simulink library "ReceiveFromGES"  (R2016b)
settings: Solver=VariableStepAuto  StartTime=0.0  StopTime=10.0  RelTol=1e-3
libraries: xpcethercatlib x12, ReceiveFromGES x3, simulink_extras x3, VariousLibrary x1
settings Model: Creator=Nathan  LastModifiedBy=march

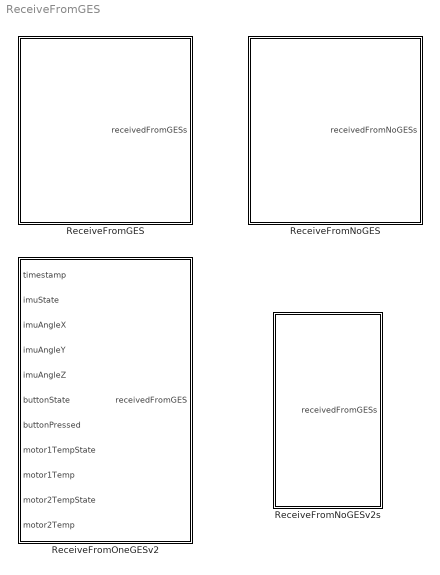
== system ReceiveFromGES ==
  ReceiveFromGES : Subsystem
  ReceiveFromNoGES : Subsystem
  ReceiveFromNoGESv2s : Subsystem
  ReceiveFromOneGESv2 : Subsystem

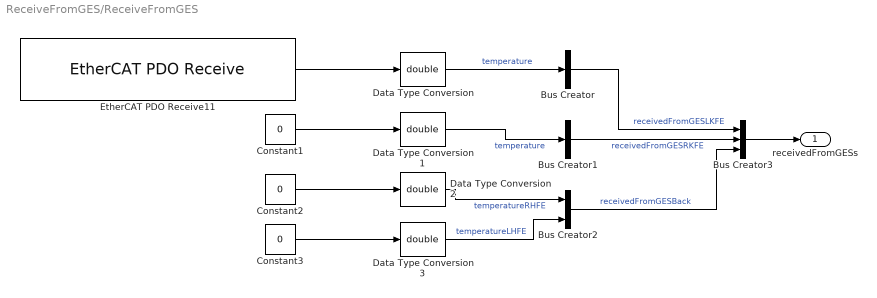
== system ReceiveFromGES/ReceiveFromGES ==
  Bus Creator : BusCreator  Inputs=1  OutDataTypeStr=Bus: EtherCATReceivedFromGESJoint  NonVirtualBus=on
  Bus Creator1 : BusCreator  Inputs=1  OutDataTypeStr=Bus: EtherCATReceivedFromGESJoint  NonVirtualBus=on
  Bus Creator2 : BusCreator  Inputs=2  OutDataTypeStr=Bus: EtherCATReceivedFromGESBack  NonVirtualBus=on
  Bus Creator3 : BusCreator  Inputs=3  OutDataTypeStr=Bus: EtherCATReceivedFromGES  NonVirtualBus=on
  Constant1 : Constant  Value=0
  Constant2 : Constant  Value=0
  Constant3 : Constant  Value=0
  Data Type Conversion{,1..3} (4 alike) : DataTypeConversion  OutDataTypeStr=double
  EtherCAT PDO Receive11 : xpcethercatlib/EtherCAT PDO Receive  Priority=2  sig_name=Box 2 (EasyCAT 32+32 configurable PDO).Inputs.temperature  sig_offset=728  sig_type=single  type_size=32  sig_dim=1  device_id=0  sample_time=0.002000
  receivedFromGESs : Outport  OutDataTypeStr=Bus: EtherCATReceivedFromGES
  wires:
  Data Type Conversion3/1 -> Bus Creator2/2  "temperatureLHFE"
  Bus Creator3/1 -> receivedFromGESs/1
  Bus Creator/1 -> Bus Creator3/1  "receivedFromGESLKFE"
  Bus Creator2/1 -> Bus Creator3/3  "receivedFromGESBack"
  Bus Creator1/1 -> Bus Creator3/2  "receivedFromGESRKFE"
  Data Type Conversion/1 -> Bus Creator/1  "temperature"
  Data Type Conversion2/1 -> Bus Creator2/1  "temperatureRHFE"
  Data Type Conversion1/1 -> Bus Creator1/1  "temperature"
  Constant1/1 -> Data Type Conversion1/1
  Constant2/1 -> Data Type Conversion2/1
  Constant3/1 -> Data Type Conversion3/1
  EtherCAT PDO Receive11/1 -> Data Type Conversion/1

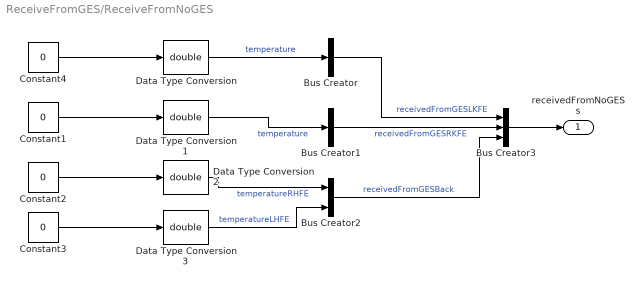
== system ReceiveFromGES/ReceiveFromNoGES ==
  Bus Creator : BusCreator  Inputs=1  OutDataTypeStr=Bus: EtherCATReceivedFromGESJoint  NonVirtualBus=on
  Bus Creator1 : BusCreator  Inputs=1  OutDataTypeStr=Bus: EtherCATReceivedFromGESJoint  NonVirtualBus=on
  Bus Creator2 : BusCreator  Inputs=2  OutDataTypeStr=Bus: EtherCATReceivedFromGESBack  NonVirtualBus=on
  Bus Creator3 : BusCreator  Inputs=3  OutDataTypeStr=Bus: EtherCATReceivedFromGES  NonVirtualBus=on
  Constant{1..4} (4 alike) : Constant  Value=0
  Data Type Conversion{,1..3} (4 alike) : DataTypeConversion  OutDataTypeStr=double
  receivedFromNoGESs : Outport  OutDataTypeStr=Bus: EtherCATReceivedFromGES
  wires:
  Constant4/1 -> Data Type Conversion/1
  Constant3/1 -> Data Type Conversion3/1
  Constant2/1 -> Data Type Conversion2/1
  Constant1/1 -> Data Type Conversion1/1
  Data Type Conversion1/1 -> Bus Creator1/1  "temperature"
  Data Type Conversion2/1 -> Bus Creator2/1  "temperatureRHFE"
  Data Type Conversion/1 -> Bus Creator/1  "temperature"
  Bus Creator1/1 -> Bus Creator3/2  "receivedFromGESRKFE"
  Bus Creator2/1 -> Bus Creator3/3  "receivedFromGESBack"
  Bus Creator/1 -> Bus Creator3/1  "receivedFromGESLKFE"
  Bus Creator3/1 -> receivedFromNoGESs/1
  Data Type Conversion3/1 -> Bus Creator2/2  "temperatureLHFE"

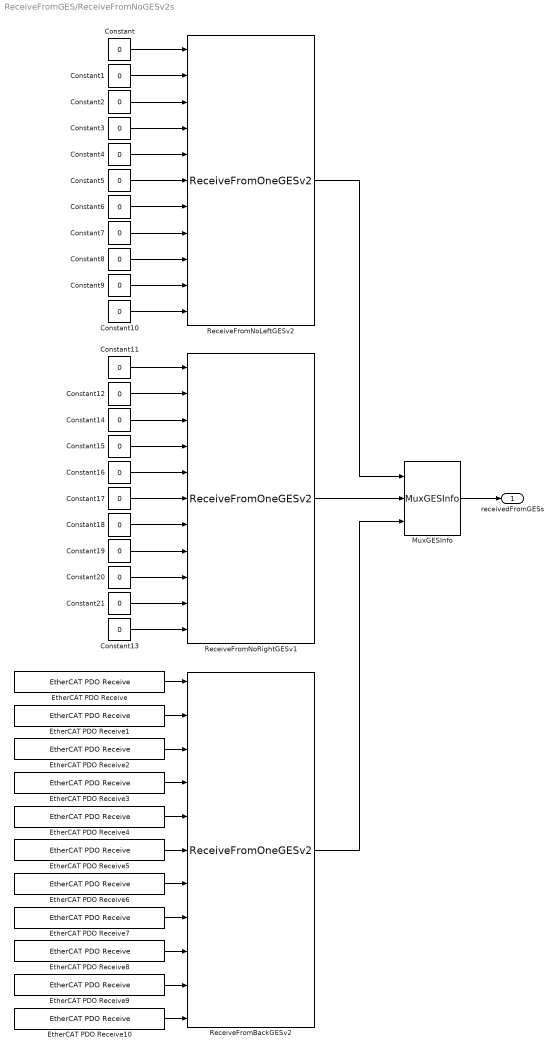
== system ReceiveFromGES/ReceiveFromNoGESv2s ==
  Constant{,1..21} (22 alike) : Constant  Value=0
  EtherCAT PDO Receive : xpcethercatlib/EtherCAT PDO Receive  Priority=2  sig_name=GES Buzzer.Inputs.heartbeat  sig_offset=632  sig_type=uint8  type_size=8  sig_dim=1  device_id=0  sample_time=0.002
  EtherCAT PDO Receive1 : xpcethercatlib/EtherCAT PDO Receive  Priority=2  sig_name=GES Buzzer.Inputs.imuEnabled  sig_offset=640  sig_type=uint8  type_size=8  sig_dim=1  device_id=0  sample_time=0.002
  EtherCAT PDO Receive10 : xpcethercatlib/EtherCAT PDO Receive  Priority=2  sig_name=GES Buzzer.Inputs.motor2Temp  sig_offset=712  sig_type=uint8  type_size=8  sig_dim=1  device_id=0  sample_time=0.002
  EtherCAT PDO Receive2 : xpcethercatlib/EtherCAT PDO Receive  Priority=2  sig_name=GES Buzzer.Inputs.imuAngleX  sig_offset=648  sig_type=uint8  type_size=8  sig_dim=1  device_id=0  sample_time=0.002
  EtherCAT PDO Receive3 : xpcethercatlib/EtherCAT PDO Receive  Priority=2  sig_name=GES Buzzer.Inputs.imuAngleY  sig_offset=656  sig_type=uint8  type_size=8  sig_dim=1  device_id=0  sample_time=0.002
  EtherCAT PDO Receive4 : xpcethercatlib/EtherCAT PDO Receive  Priority=2  sig_name=GES Buzzer.Inputs.imuAngleZ  sig_offset=664  sig_type=uint8  type_size=8  sig_dim=1  device_id=0  sample_time=0.002
  EtherCAT PDO Receive5 : xpcethercatlib/EtherCAT PDO Receive  Priority=2  sig_name=GES Buzzer.Inputs.buttonEnabled  sig_offset=672  sig_type=uint8  type_size=8  sig_dim=1  device_id=0  sample_time=0.002
  EtherCAT PDO Receive6 : xpcethercatlib/EtherCAT PDO Receive  Priority=2  sig_name=GES Buzzer.Inputs.buttonState  sig_offset=680  sig_type=uint8  type_size=8  sig_dim=1  device_id=0  sample_time=0.002
  EtherCAT PDO Receive7 : xpcethercatlib/EtherCAT PDO Receive  Priority=2  sig_name=GES Buzzer.Inputs.motor1TempEnabled  sig_offset=688  sig_type=uint8  type_size=8  sig_dim=1  device_id=0  sample_time=0.002
  EtherCAT PDO Receive8 : xpcethercatlib/EtherCAT PDO Receive  Priority=2  sig_name=GES Buzzer.Inputs.motor1Temp  sig_offset=704  sig_type=uint8  type_size=8  sig_dim=1  device_id=0  sample_time=0.002
  EtherCAT PDO Receive9 : xpcethercatlib/EtherCAT PDO Receive  Priority=2  sig_name=GES Buzzer.Inputs.motor2TempEnabled  sig_offset=696  sig_type=uint8  type_size=8  sig_dim=1  device_id=0  sample_time=0.002
  MuxGESInfo : VariousLibrary/MuxGESInfo
  ReceiveFromBackGESv2 : ReceiveFromGES/ReceiveFromOneGESv2
  ReceiveFromNoLeftGESv2 : ReceiveFromGES/ReceiveFromOneGESv2
  ReceiveFromNoRightGESv1 : ReceiveFromGES/ReceiveFromOneGESv2
  receivedFromGESs : Outport
  wires:
  EtherCAT PDO Receive10/1 -> ReceiveFromBackGESv2/11
  EtherCAT PDO Receive9/1 -> ReceiveFromBackGESv2/10
  EtherCAT PDO Receive8/1 -> ReceiveFromBackGESv2/9
  EtherCAT PDO Receive7/1 -> ReceiveFromBackGESv2/8
  EtherCAT PDO Receive6/1 -> ReceiveFromBackGESv2/7
  EtherCAT PDO Receive5/1 -> ReceiveFromBackGESv2/6
  EtherCAT PDO Receive4/1 -> ReceiveFromBackGESv2/5
  EtherCAT PDO Receive3/1 -> ReceiveFromBackGESv2/4
  EtherCAT PDO Receive2/1 -> ReceiveFromBackGESv2/3
  EtherCAT PDO Receive1/1 -> ReceiveFromBackGESv2/2
  EtherCAT PDO Receive/1 -> ReceiveFromBackGESv2/1
  Constant/1 -> ReceiveFromNoLeftGESv2/1
  Constant1/1 -> ReceiveFromNoLeftGESv2/2
  Constant4/1 -> ReceiveFromNoLeftGESv2/5
  Constant2/1 -> ReceiveFromNoLeftGESv2/3
  Constant5/1 -> ReceiveFromNoLeftGESv2/6
  Constant10/1 -> ReceiveFromNoLeftGESv2/11
  Constant7/1 -> ReceiveFromNoLeftGESv2/8
  Constant3/1 -> ReceiveFromNoLeftGESv2/4
  Constant6/1 -> ReceiveFromNoLeftGESv2/7
  Constant8/1 -> ReceiveFromNoLeftGESv2/9
  Constant9/1 -> ReceiveFromNoLeftGESv2/10
  Constant11/1 -> ReceiveFromNoRightGESv1/1
  Constant12/1 -> ReceiveFromNoRightGESv1/2
  Constant16/1 -> ReceiveFromNoRightGESv1/5
  Constant14/1 -> ReceiveFromNoRightGESv1/3
  Constant17/1 -> ReceiveFromNoRightGESv1/6
  Constant13/1 -> ReceiveFromNoRightGESv1/11
  Constant19/1 -> ReceiveFromNoRightGESv1/8
  Constant15/1 -> ReceiveFromNoRightGESv1/4
  Constant18/1 -> ReceiveFromNoRightGESv1/7
  Constant20/1 -> ReceiveFromNoRightGESv1/9
  Constant21/1 -> ReceiveFromNoRightGESv1/10
  ReceiveFromNoRightGESv1/1 -> MuxGESInfo/2
  ReceiveFromNoLeftGESv2/1 -> MuxGESInfo/1
  ReceiveFromBackGESv2/1 -> MuxGESInfo/3
  MuxGESInfo/1 -> receivedFromGESs/1

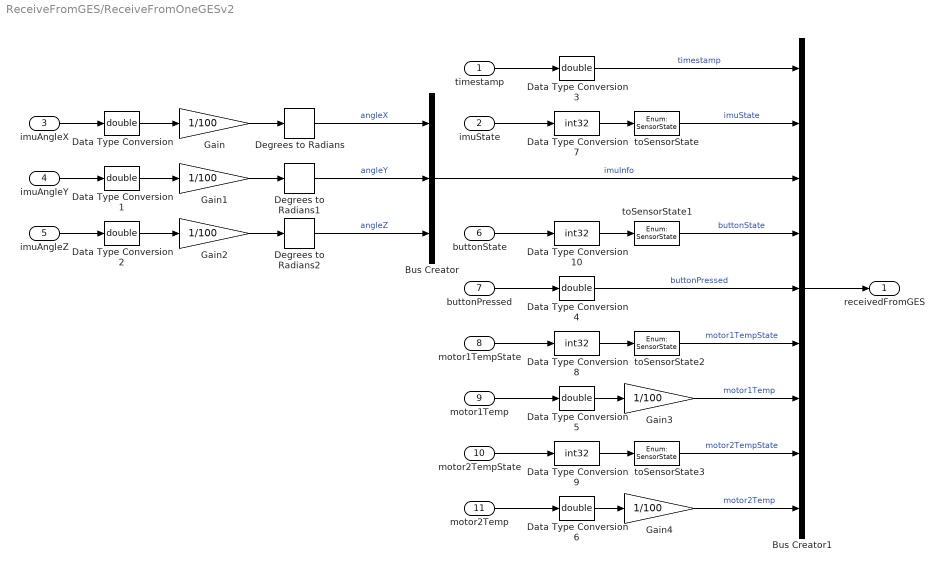
== system ReceiveFromGES/ReceiveFromOneGESv2 ==
  timestamp : Inport
  imuState : Inport  Port=2
  imuAngleX : Inport  Port=3
  imuAngleY : Inport  Port=4
  imuAngleZ : Inport  Port=5
  buttonState : Inport  Port=6
  buttonPressed : Inport  Port=7
  motor1TempState : Inport  Port=8
  motor1Temp : Inport  Port=9
  motor2TempState : Inport  Port=10
  motor2Temp : Inport  Port=11
  Bus Creator : BusCreator  Inputs=3  OutDataTypeStr=Bus: IMUInfo  NonVirtualBus=on
  Bus Creator1 : BusCreator  Inputs=9  OutDataTypeStr=Bus: EtherCATReceivedFromGES  NonVirtualBus=on
  Data Type Conversion{,1..6} (7 alike) : DataTypeConversion  OutDataTypeStr=double
  Data Type Conversion{7..10} (4 alike) : DataTypeConversion  OutDataTypeStr=int32
  Degrees to Radians : simulink_extras/Transformations/Degrees to Radians
  Degrees to Radians1 : simulink_extras/Transformations/Degrees to Radians
  Degrees to Radians2 : simulink_extras/Transformations/Degrees to Radians
  Gain{,1..4} (5 alike) : Gain  Gain=1/100
  toSensorState{,1..3} (4 alike) : DataTypeConversion  OutDataTypeStr=Enum: SensorState  RndMeth=Nearest
  receivedFromGES : Outport
  wires:
  Data Type Conversion10/1 -> toSensorState1/1
  Data Type Conversion9/1 -> toSensorState3/1
  Data Type Conversion8/1 -> toSensorState2/1
  Data Type Conversion7/1 -> toSensorState/1
  timestamp/1 -> Data Type Conversion3/1
  imuState/1 -> Data Type Conversion7/1
  Bus Creator/1 -> Bus Creator1/3  "imuInfo"
  motor2TempState/1 -> Data Type Conversion9/1
  buttonPressed/1 -> Data Type Conversion4/1
  motor1TempState/1 -> Data Type Conversion8/1
  motor1Temp/1 -> Data Type Conversion5/1
  motor2Temp/1 -> Data Type Conversion6/1
  buttonState/1 -> Data Type Conversion10/1
  Data Type Conversion/1 -> Gain/1
  imuAngleX/1 -> Data Type Conversion/1
  Degrees to Radians/1 -> Bus Creator/1  "angleX"
  imuAngleY/1 -> Data Type Conversion1/1
  Data Type Conversion1/1 -> Gain1/1
  Degrees to Radians1/1 -> Bus Creator/2  "angleY"
  imuAngleZ/1 -> Data Type Conversion2/1
  Data Type Conversion2/1 -> Gain2/1
  Degrees to Radians2/1 -> Bus Creator/3  "angleZ"
  Data Type Conversion3/1 -> Bus Creator1/1  "timestamp"
  Gain/1 -> Degrees to Radians/1
  Gain1/1 -> Degrees to Radians1/1
  Gain2/1 -> Degrees to Radians2/1
  toSensorState/1 -> Bus Creator1/2  "imuState"
  toSensorState1/1 -> Bus Creator1/4  "buttonState"
  toSensorState2/1 -> Bus Creator1/6  "motor1TempState"
  toSensorState3/1 -> Bus Creator1/8  "motor2TempState"
  Bus Creator1/1 -> receivedFromGES/1
  Data Type Conversion4/1 -> Bus Creator1/5  "buttonPressed"
  Data Type Conversion5/1 -> Gain3/1
  Data Type Conversion6/1 -> Gain4/1
  Gain3/1 -> Bus Creator1/7  "motor1Temp"
  Gain4/1 -> Bus Creator1/9  "motor2Temp"
